simulink model "InsertedEarbud"  (R2024a)
settings: Solver=daessc  StartTime=0.0  StopTime=T  RelTol=1e-3
model workspace (MAT data in the model file):
  Nbud = Simulink.Parameter
  Nbud.Value = 1
  Nbud.Complexity = 'real'
  Nbud.Dimensions = [1 1]
  Nbud.Description = 'number of sound holes on earbud cavity'
  Nbud.DataType = 'auto'
  Nf = Simulink.Parameter
  Nf.Value = 18
  Nf.Complexity = 'real'
  Nf.Dimensions = [1 1]
  Nf.Description = 'Number of front cover holes (guess)'
  Nf.DataType = 'auto'
  Nv = Simulink.Parameter
  Nv.Value = 4
  Nv.Complexity = 'real'
  Nv.Dimensions = [1 1]
  Nv.Description = 'Number of vent holes (guess)'
  Nv.DataType = 'auto'
  T = Simulink.Parameter
  T.Value = 3
  T.Complexity = 'real'
  T.Dimensions = [1 1]
  T.Description = 'simulation time '
  T.DataType = 'auto'
  Vb = Simulink.Parameter
  Vb.Value = 5.0877e-08
  Vb.Complexity = 'real'
  Vb.Dimensions = [1 1]
  Vb.Description = 'Rear cavity of microspeaker (estimated)'
  Vb.DataType = 'auto'
  Vb.DocUnits = 'm^3'
  Vbud = Simulink.Parameter
  Vbud.Value = 2.4811e-07
  Vbud.Complexity = 'real'
  Vbud.Dimensions = [1 1]
  Vbud.Description = 'earbud rear cavity volume (estimated)'
  Vbud.DataType = 'auto'
  Vbud.DocUnits = 'm^3'
  Vf = Simulink.Parameter
  Vf.Value = 5.1281e-08
  Vf.Complexity = 'real'
  Vf.Dimensions = [1 1]
  Vf.Description = 'Front cavity volume of microspeaker (estimated)'
  Vf.DataType = 'auto'
  Vf.DocUnits = 'm^3 '
  c = Simulink.Parameter
  c.Value = 343
  c.Complexity = 'real'
  c.Dimensions = [1 1]
  c.Description = 'sound speed in air'
  c.DataType = 'auto'
  c.DocUnits = 'm/s'
  dt = Simulink.Parameter
  dt.Value = 2.26757369615e-05
  dt.Complexity = 'real'
  dt.Dimensions = [1 1]
  dt.Description = 'sampling time '
  dt.DataType = 'auto'
  fix_l = Simulink.Parameter
  fix_l.Value = 0.0066
  fix_l.Complexity = 'real'
  fix_l.Dimensions = [1 1]
  fix_l.Description = 'fixture tube length'
  fix_l.DataType = 'auto'
  fix_l.DocUnits = 'm'
  fix_r = Simulink.Parameter
  fix_r.Value = 0.0037
  fix_r.Complexity = 'real'
  fix_r.Dimensions = [1 1]
  fix_r.Description = 'fixture tube radius'
  fix_r.DataType = 'auto'
  fix_r.DocUnits = 'm'
  lbud = Simulink.Parameter
  lbud.Value = 0.12
  lbud.Complexity = 'real'
  lbud.Dimensions = [1 1]
  lbud.Description = 'earbud rear vent thickness'
  lbud.DataType = 'auto'
  lbud.DocUnits = 'm'
  leak_A = Simulink.Parameter
  leak_A.Value = Simulink.data.Expression
  leak_A.Value.ExpressionString = "leak_r^2*pi"
  leak_A.Complexity = 'real'
  leak_A.Dimensions = -1
  leak_A.Description = 'earbud front vent area'
  leak_A.DataType = 'auto'
  leak_A.DocUnits = 'm^2'
  leak_l = Simulink.Parameter
  leak_l.Value = 0.001
  leak_l.Complexity = 'real'
  leak_l.Dimensions = [1 1]
  leak_l.Description = 'earbud front vent length'
  leak_l.DataType = 'auto'
  leak_l.DocUnits = 'm'
  leak_r = Simulink.Parameter
  leak_r.Value = 9.7721e-05
  leak_r.Complexity = 'real'
  leak_r.Dimensions = [1 1]
  leak_r.Description = 'earbud front vent radius'
  leak_r.DataType = 'auto'
  leak_r.DocUnits = 'm'
  nu = Simulink.Parameter
  nu.Value = 1.568e-05
  nu.Complexity = 'real'
  nu.Dimensions = [1 1]
  nu.Description = 'air kinematice viscousity'
  nu.DataType = 'auto'
  nu.DocUnits = 'm^2/s'
  rbud = Simulink.Parameter
  rbud.Value = 0.005
  rbud.Complexity = 'real'
  rbud.Dimensions = [1 1]
  rbud.Description = 'earbud rear vent radius'
  rbud.DataType = 'auto'
  rbud.DocUnits = 'm'
  rf = Simulink.Parameter
  rf.Value = 0.0005
  rf.Complexity = 'real'
  rf.Dimensions = [1 1]
  rf.Description = 'Front cover holes radius of the speaker'
  rf.DataType = 'auto'
  rf.DocUnits = 'm'
  rho = Simulink.Parameter
  rho.Value = 1.21
  rho.Complexity = 'real'
  rho.Dimensions = [1 1]
  rho.Description = 'air density'
  rho.DataType = 'auto'
  rho.DocUnits = 'kg/m^3'
  rv = Simulink.Parameter
  rv.Value = 0.000205
  rv.Complexity = 'real'
  rv.Dimensions = [1 1]
  rv.Description = 'vent radius (estimated) of the speaker'
  rv.DataType = 'auto'
  rv.DocUnits = 'm'
  spk_A = Simulink.Parameter
  spk_A.Value = Simulink.data.Expression
  spk_A.Value.ExpressionString = "spk_r^2*pi"
  spk_A.Complexity = 'real'
  spk_A.Dimensions = -1
  spk_A.Description = 'speaker diaphragm area'
  spk_A.DataType = 'auto'
  spk_A.DocUnits = 'm^2 '
  spk_d = Simulink.Parameter
  spk_d.Value = 0.009
  spk_d.Complexity = 'real'
  spk_d.Dimensions = [1 1]
  spk_d.Description = 'speaker diameter'
  spk_d.DataType = 'auto'
  spk_d.DocUnits = 'm'
  spk_r = Simulink.Parameter
  spk_r.Value = Simulink.data.Expression
  spk_r.Value.ExpressionString = "spk_d/2"
  spk_r.Complexity = 'real'
  spk_r.Dimensions = -1
  spk_r.Description = 'speaker radius'
  spk_r.DataType = 'auto'
  spk_r.DocUnits = 'm'
  thikf = Simulink.Parameter
  thikf.Value = 0.0003
  thikf.Complexity = 'real'
  thikf.Dimensions = [1 1]
  thikf.Description = 'Front cover holes thickness of the speaker'
  thikf.DataType = 'auto'
  thikf.DocUnits = 'm'
  thikv = Simulink.Parameter
  thikv.Value = 0.00025
  thikv.Complexity = 'real'
  thikv.Dimensions = [1 1]
  thikv.Description = 'vent length of the speaker'
  thikv.DataType = 'auto'
  thikv.DocUnits = 'm'
  tip_l = Simulink.Parameter
  tip_l.Value = 0.005
  tip_l.Complexity = 'real'
  tip_l.Dimensions = [1 1]
  tip_l.Description = 'earbud tip length'
  tip_l.DataType = 'auto'
  tip_l.DocUnits = 'm'
  tip_r = Simulink.Parameter
  tip_r.Value = 0.0025
  tip_r.Complexity = 'real'
  tip_r.Dimensions = [1 1]
  tip_r.Description = 'earbud tip radius'
  tip_r.DataType = 'auto'
  tip_r.DocUnits = 'm'
  tube_l = Simulink.Parameter
  tube_l.Value = 0.0053
  tube_l.Complexity = 'real'
  tube_l.Dimensions = [1 1]
  tube_l.Description = 'earbud sound tube length'
  tube_l.DataType = 'auto'
  tube_l.DocUnits = 'm'
  tube_r = Simulink.Parameter
  tube_r.Value = 0.002
  tube_r.Complexity = 'real'
  tube_r.Dimensions = [1 1]
  tube_r.Description = 'earbud sound tube radius '
  tube_r.DataType = 'auto'
  tube_r.DocUnits = 'm'
undefined symbols (not defined in the file): acoustic
libraries: acoustic_lib x8, fl_lib x3, nesl_utility x3, simulink x1
settings Model: Creator=andychen  LastModifiedBy=ftiong
settings DataIOCC: OutputOption=SpecifiedOutputTimes  OutputTimes=0:dt:T

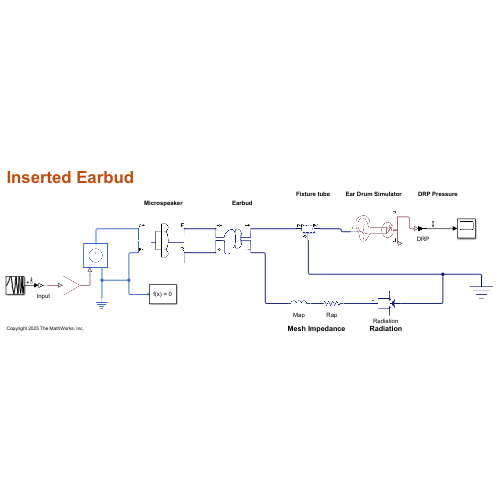
[thumbnail: Simulink's stored preview of the top-level diagram]
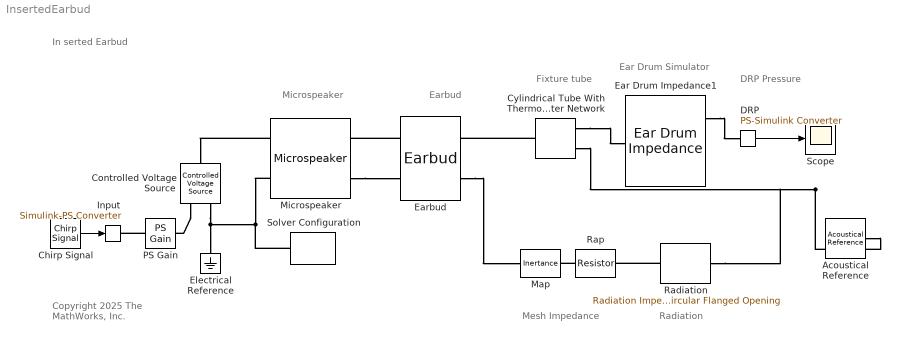
== system InsertedEarbud ==
  note: Copyright 2025 The MathWorks, Inc.
  note: Radiation
  note: Fixture tube
  note: Ear Drum Simulator
  note: Mesh Impedance
  note: DRP Pressure
  note: Earbud
  note: Microspeaker
  note: In serted Earbud
  Acoustical Reference : acoustic_lib/Acoustical Elements/Acoustical Reference
      settings: SourceProductName=Acoustic  InternalSimscapePortConfiguration="{\"Bottom\":[],\"Left\":[],\"Right\":[],\"Top\":[{\"id\":\"pp\",\"label\":\"\",\"type\":\"acoustic.acoustic\"}]}"
  Chirp Signal : simulink/Sources/Chirp Signal  f1=10  T=T  f2=20e3
  Controlled Voltage Source : fl_lib/Electrical/Electrical Sources/Controlled Voltage Source
  Cylindrical Tube With Thermoviscous Losses Using Foster Network : acoustic_lib/Applications/Tubes and Horns/Cylindrical Tube With Thermoviscous Losses Using Foster Network  a=fix_r m  length=fix_l m  mdl=acoustic.enum.Tubemdl.simple  order=4  Ndl=20
      settings: SourceProductName=Acoustic  InternalSimscapePortConfiguration="{\"Bottom\":[{\"id\":\"p3\",\"label\":\"P3\",\"type\":\"acoustic.acoustic\"}],\"Left\":[{\"id\":\"p1\",\"label\":\"P1\",\"type\":\"acoustic.acoustic\"}],\"Right\":[{\"id\":\"p2\",\"label\":\"P2\",\"type\":\"acoustic.acoustic\"}],\"Top\":[]}"
  DRP : nesl_utility/PS-Simulink Converter  PhysicalDomain=network_engine_domain  SubClassName=ps_output  LeftPortType=input  RightPortType=output  PseudoPeriodic=off  Frequencies=[]  VectorFormat=inherit  Unit=inherit  AffineConversion=off
  Ear Drum Impedance1 : acoustic_lib/Applications/Human Ear/Ear Drum Impedance  Ma1=82.9 Pa*s^2/m^3  Ma2=9400 Pa*s^2/m^3  Ma3=130.3 Pa*s^2/m^3  Ma4=983.8 Pa*s^2/m^3  Ma5=133.4 Pa*s^2/m^3  Ca1=0.7e-12 m^3/Pa  Ca2=2.34e-12 m^3/Pa  Ca3=1.5e-12 m^3/Pa  Ca4=2.73e-12 m^3/Pa  Ca5=1.517e-12 m^3/Pa  Ra2=55.66e6 Pa*s/m^3  Ra4=27.99e6 Pa*s/m^3  damping1=acoustic.enum.R1.includeR1  damping3=acoustic.enum.R3.includeR3  damping5=acoustic.enum.R5.includeR5  Ra1=4.22e5 Pa*s/m^3  Ra3=4.22e5 Pa*s/m^3  Ra5=3.22e6 Pa*s/m^3
      settings: SourceProductName=Acoustic  InternalSimscapePortConfiguration="{\"Bottom\":[],\"Left\":[{\"id\":\"pa\",\"label\":\"+\",\"type\":\"acoustic.acoustic\"}],\"Right\":[{\"id\":\"P\",\"label\":\"P\",\"type\":\"output\"},{\"id\":\"U\",\"label\":\"U\",\"type\":\"output\"}],\"Top\":[]}"
  Earbud : acoustic_lib/Applications/Headphones/Earbud  tube_earbud=acoustic.enum.Bud_Tube.include_tube  tube_l=tube_l m  tube_r=tube_r m  tip_earbud=acoustic.enum.Bud_Tip.include_tip  tip_l=tip_l m  tip_r=tip_r m  fvent_earbud=acoustic.enum.Bud_FrontVent(2)  fvent_l=leak_l m  fvent_r=leak_r m  Nfv_bud=1  rvent_earbud=acoustic.enum.Bud_RearVent(2)  rvent_l=lbud m  rvent_r=rbud m  Nrv_bud=1  frvent_earbud=acoustic.enum.Bud_FRVent.without_front_to_rear  frvent_l=0.001 m  frvent_r=9.7721e-04 m  Nfr_bud=1  leakage=acoustic.enum.Bud_Leak.include_leak  leak_l=leak_l*5e-1 m  leak_r=leak_r*1e-1 m  bud_Vb=Vbud m^3
      settings: SourceProductName=Acoustic  InternalSimscapePortConfiguration="{\"Bottom\":[],\"Left\":[{\"id\":\"pb\",\"label\":\"R+\",\"type\":\"acoustic.acoustic\"},{\"id\":\"nb\",\"label\":\"R-\",\"type\":\"acoustic.acoustic\"}],\"Right\":[{\"id\":\"pf\",\"label\":\"F+\",\"type\":\"acoustic.acoustic\"},{\"id\":\"nf\",\"label\":\"F-\",\"type\":\"acoustic.acoustic\"}],\"Top\":[]}"
  Electrical Reference : fl_lib/Electrical/Electrical Elements/Electrical Reference
  Input : nesl_utility/Simulink-PS Converter  PhysicalDomain=network_engine_domain  SubClassName=ps_input  LeftPortType=input  RightPortType=output  PseudoPeriodic=off  Frequencies=[]  NoiseDistribution=none  NoiseParameters=[]  Unit=1  AffineConversion=off  FilteringAndDerivatives=provide  SimscapeFilterOrder=1  InputFilterTimeConstant=0.001  UdotUserProvided=0
  Map : acoustic_lib/Acoustical Elements/Inertance  m=0.01 Pa*s^2/m^3  r_m=1e-9 Pa*s/m^3  g_m=1e-9 m^3/(Pa*s)  u_specify=off  u_priority=None  u=0 m^3/s  u_nominal_specify=off  u_nominal_value=1  u_nominal_unit=m^3/s  p_specify=off  p_priority=None  p=0 Pa  p_nominal_specify=off  p_nominal_value=1  p_nominal_unit=Pa  U_m_specify=off  U_m_priority=High  U_m=0 m^3/s  U_m_nominal_specify=off  U_m_nominal_value=1  U_m_nominal_unit=m^3/s
      settings: SourceProductName=Acoustic  InternalSimscapePortConfiguration="{\"Bottom\":[],\"Left\":[{\"id\":\"pp\",\"label\":\"+\",\"type\":\"acoustic.acoustic\"}],\"Right\":[{\"id\":\"nn\",\"label\":\"-\",\"type\":\"acoustic.acoustic\"}],\"Top\":[]}"
  Microspeaker : acoustic_lib/Applications/Moving Coil Speakers/Microspeaker  Re=31.14 Ohm  Le=14e-5 H  Bl=0.719 N/A  Mm=23e-6 kg  Km=1 / 25.12e-3 N/m  Rm=3e-3 kg/s  Sd=0.0001271 m^2  Vb=1.01646e-7 m^3  thikv=0.0005 m  rv=0.00041 m  Nv=8  tmesh=2.43e-14 m  rmesh=9.6755e-7 m  frontCov=acoustic.enum.MicroSPK_FrontCov.include_front_cover  Vf=1.02453e-7 m^3  thikf=0.0003 m  rf=0.0005 m  Nf=36
      settings: SourceProductName=Acoustic  InternalSimscapePortConfiguration="{\"Bottom\":[],\"Left\":[{\"id\":\"pe\",\"label\":\"e+\",\"type\":\"foundation.electrical.electrical\"},{\"id\":\"ne\",\"label\":\"e-\",\"type\":\"foundation.electrical.electrical\"}],\"Right\":[{\"id\":\"pa\",\"label\":\"F\",\"type\":\"acoustic.acoustic\"},{\"id\":\"na\",\"label\":\"R\",\"type\":\"acoustic.acoustic\"}],\"Top\":[]}"
  PS Gain : fl_lib/Physical Signals/Functions/PS Gain  gain=0.179 V
  Radiation : acoustic_lib/Radiation Impedance/Radiation Impedance - Circular Flanged Opening  r=rbud m
      settings: SourceProductName=Acoustic  InternalSimscapePortConfiguration="{\"Bottom\":[],\"Left\":[{\"id\":\"pa\",\"label\":\"+\",\"type\":\"acoustic.acoustic\"}],\"Right\":[{\"id\":\"na\",\"label\":\"-\",\"type\":\"acoustic.acoustic\"}],\"Top\":[]}"
  Rap : acoustic_lib/Acoustical Elements/Resistor  R_r=5.84e8 Pa*s/m^3  u_specify=off  u_priority=None  u=0 m^3/s  u_nominal_specify=off  u_nominal_value=1  u_nominal_unit=m^3/s  p_specify=off  p_priority=None  p=0 Pa  p_nominal_specify=off  p_nominal_value=1  p_nominal_unit=Pa
      settings: SourceProductName=Acoustic  InternalSimscapePortConfiguration="{\"Bottom\":[],\"Left\":[{\"id\":\"pp\",\"label\":\"+\",\"type\":\"acoustic.acoustic\"}],\"Right\":[{\"id\":\"nn\",\"label\":\"-\",\"type\":\"acoustic.acoustic\"}],\"Top\":[]}"
  Scope : Scope
  Solver Configuration : nesl_utility/Solver Configuration  PhysicalDomain=network_engine_domain  SubClassName=solver  LeftPortType=input  RightPortType=generic  Tones=[]  Harmonics=[]  SimulateNoise=off  Profile=off  UseLocalSampling=off  EnableSwitchedLinearOptims=on  FrequencyDomain=off  UseCCode=off  RelTol=0.001  AbsTol=0.001  MinStep=1e-09  ToWorkspace=off  RevertToSquareIcSolve=off  NumHomotopyIterations=100  PhasorMode=off  PhasorModeNumHarmonics=1  ConsistencySolver=NEWTON_XTOL_AFTER_FTOL  IndexReductionMethod=DerivativeReplacement  DoDC=off  ResidualTolerance=1e-09  ConsistencyTolSource=GLOBAL  ConsistencyAbsTol=0.001  ConsistencyRelTol=0.001  ConsistencyTolFactor=0.001  UseLocalSolver=off  LocalSolverChoice=NE_BACKWARD_EULER_ADVANCER  ResolveIndetEquations=on  FunctionEvalNumThread=1  LocalSolverSampleTime=0.001  DoFixedCost=off  MaxNonlinIter=3  MaxModeIter=2  ComputeImpulses=off  ImpulseIterations=2  LinearAlgebra=auto  LinearAlgebraNumThread=0  EquationFormulation=NE_TIME_EF  DelaysMemoryBudget=1024  AutomaticFiltering=on  FilteringTimeConstant=0.001  PartitionStorageMethod=AS_NEEDED  PartitionMemoryBudget=1024  PartitionMethod=ROBUST  MultibodyUseLocalSolver=off  MultibodyLocalSolverChoice=ODE1  MultibodyLocalSolverSampleTime=0.001
  wires:
  Chirp Signal/1 -> Input/1
  DRP/1 -> Scope/1
  connections:
  PS Gain/LConn1 -- Input/RConn1
  Controlled Voltage Source/RConn1 -- PS Gain/RConn1
  Microspeaker/LConn1 -- Controlled Voltage Source/LConn1
  Cylindrical Tube With Thermoviscous Losses Using Foster Network/RConn1 -- Ear Drum Impedance1/LConn1
  Rap/LConn1 -- Map/RConn1
  Radiation/LConn1 -- Rap/RConn1
  Cylindrical Tube With Thermoviscous Losses Using Foster Network/RConn2 -- Radiation/RConn1 -- Acoustical Reference/LConn1
  Cylindrical Tube With Thermoviscous Losses Using Foster Network/LConn1 -- Earbud/RConn1
  Microspeaker/RConn2 -- Earbud/LConn2
  Earbud/LConn1 -- Microspeaker/RConn1
  Earbud/RConn2 -- Map/LConn1
  Controlled Voltage Source/RConn2 -- Microspeaker/LConn2 -- Solver Configuration/RConn1 -- Electrical Reference/LConn1
  Ear Drum Impedance1/RConn1 -- DRP/LConn1
